simulink model "hybrid_system_diag"  (Simulink 7.8)
settings: Solver=FixedStepDiscrete  StartTime=0.0  StopTime=10  FixedStep=sim_sample_time  RelTol=1e-6
undefined symbols (not defined in the file or in its folder): SysHybride
settings Model: Creator=bayoudh  LastModifiedBy=szabi  ExtModeAutoUpdateStatusClock=off
settings OptimizationCC: InitFltsAndDblsToZero=on
settings DebuggingCC: SaveWithParameterizedLinksMsg=none  FcnCallInpInsideContextMsg=Use local settings  StrictBusMsg=Warning
settings SFSimCC: SimParseCustomCode=off
settings GRTTargetCC: TargetFcnLib=ansi_tfl_tmw.mat

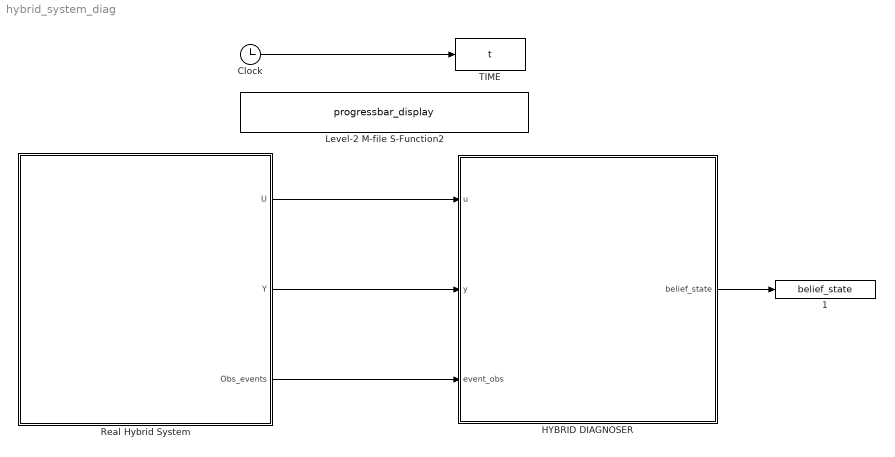
== system hybrid_system_diag ==
  1 : ToWorkspace  VariableName=belief_state  SampleTime=-1  SaveFormat=Array
  Clock : Clock
  "HYBRID DIAGNOSER " : Subsystem
  Level-2 M-file S-Function2 : M-S-Function  FunctionName=progressbar_display
  Real Hybrid System : Subsystem
  TIME : ToWorkspace  VariableName=t  SampleTime=-1  SaveFormat=Array
  wires:
  Clock/1 -> TIME/1
  Real Hybrid System/1(U) -> "HYBRID DIAGNOSER "/1(u)
  Real Hybrid System/2(Y) -> "HYBRID DIAGNOSER "/2(y)
  Real Hybrid System/3(Obs_events) -> "HYBRID DIAGNOSER "/3(event_obs)
  "HYBRID DIAGNOSER "/1(belief_state) -> 1/1

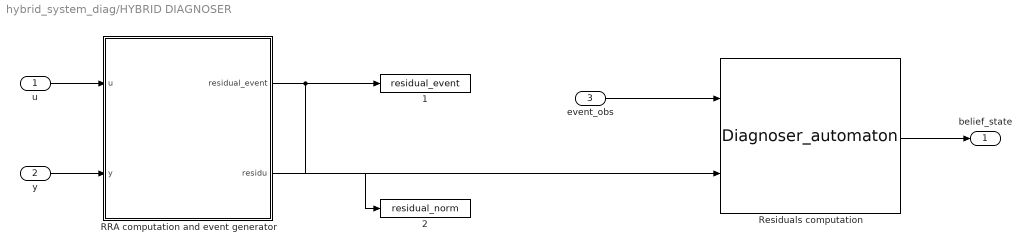
== system hybrid_system_diag/HYBRID DIAGNOSER  ==
  u : Inport
  y : Inport  Port=2
  event_obs : Inport  Port=3
  1 : ToWorkspace  VariableName=residual_event  SampleTime=-1  SaveFormat=Array
  2 : ToWorkspace  VariableName=residual_norm  SampleTime=-1  SaveFormat=Array
  RRA computation and event generator : Subsystem
  Residuals computation : M-S-Function  FunctionName=Diagnoser_automaton
  belief_state : Outport
  wires:
  u/1 -> RRA computation and event generator/1(u)
  y/1 -> RRA computation and event generator/2(y)
  RRA computation and event generator/1(residual_event) -> 1/1, Residuals computation/2
  RRA computation and event generator/2(residu) -> 2/1
  event_obs/1 -> Residuals computation/1
  Residuals computation/1 -> belief_state/1

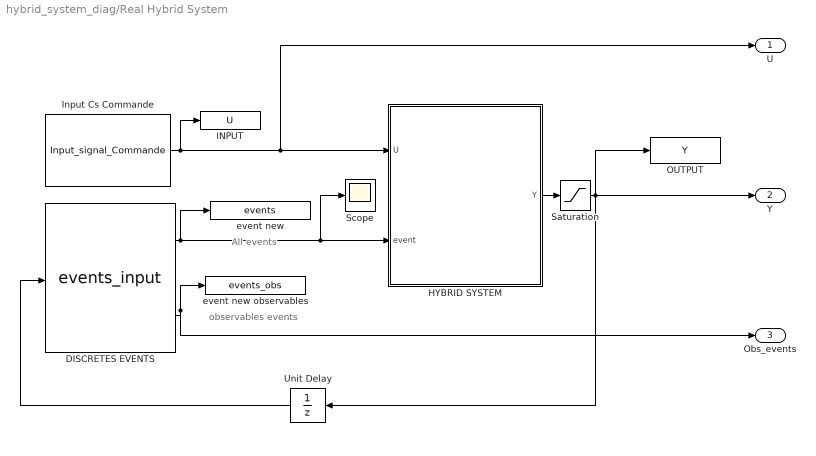
== system hybrid_system_diag/Real Hybrid System ==
  note: observables events
  note: All events
  DISCRETES EVENTS : M-S-Function  FunctionName=events_input
  HYBRID SYSTEM : Subsystem
  INPUT : ToWorkspace  VariableName=U  SampleTime=-1  SaveFormat=Array
  Input Cs Commande : S-Function  FunctionName=Input_signal_Commande  Parameters=rand(SysHybride('get_input_size'),1)*2*pi  EnableBusSupport=off
  OUTPUT : ToWorkspace  VariableName=Y  SampleTime=-1  SaveFormat=Array
  Saturation : Saturate  UpperLimit=Inf  LowerLimit=0
  Scope : Scope
  Unit Delay : UnitDelay  SampleTime=-1
  event new : ToWorkspace  VariableName=events  SampleTime=-1  SaveFormat=Array
  event new observables : ToWorkspace  VariableName=events_obs  SampleTime=-1  SaveFormat=Array
  U : Outport
  Y : Outport  Port=2
  Obs_events : Outport  Port=3
  wires:
  Input Cs Commande/1 -> INPUT/1, HYBRID SYSTEM/1(U), U/1
  HYBRID SYSTEM/1(Y) -> Saturation/1
  DISCRETES EVENTS/1 -> event new/1, HYBRID SYSTEM/2(event), Scope/1
  DISCRETES EVENTS/2 -> event new observables/1, Obs_events/1
  Unit Delay/1 -> DISCRETES EVENTS/1
  Saturation/1 -> Y/1, OUTPUT/1, Unit Delay/1

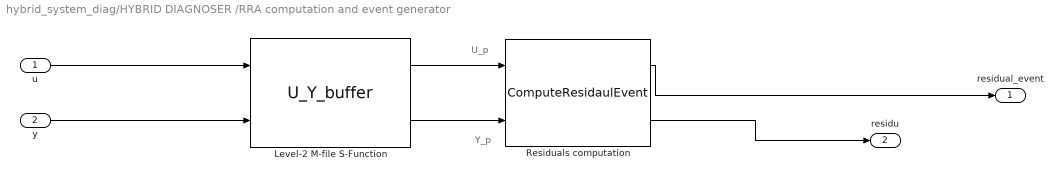
== system hybrid_system_diag/HYBRID DIAGNOSER /RRA computation and event generator ==
  note: U_p
  note: Y_p
  u : Inport
  y : Inport  Port=2
  Level-2 M-file S-Function : M-S-Function  FunctionName=U_Y_buffer
  Residuals computation : M-S-Function  FunctionName=ComputeResidaulEvent
  residual_event : Outport
  residu : Outport  Port=2
  wires:
  u/1 -> Level-2 M-file S-Function/1
  y/1 -> Level-2 M-file S-Function/2
  Level-2 M-file S-Function/1 -> Residuals computation/1
  Level-2 M-file S-Function/2 -> Residuals computation/2
  Residuals computation/1 -> residual_event/1
  Residuals computation/2 -> residu/1

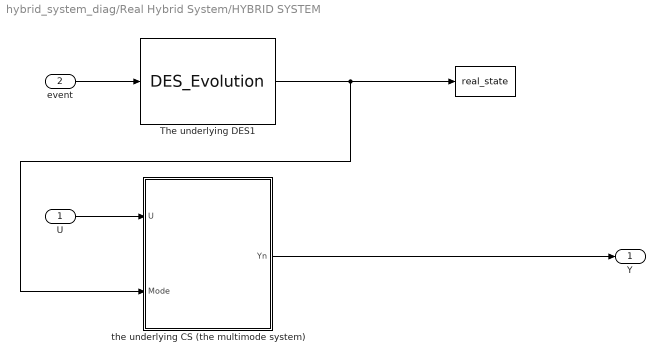
== system hybrid_system_diag/Real Hybrid System/HYBRID SYSTEM ==
  U : Inport
  event : Inport  Port=2
  "  " : ToWorkspace  VariableName=real_state  SampleTime=-1  SaveFormat=Array
  The underlying DES1 : S-Function  FunctionName=DES_Evolution  EnableBusSupport=off
  the underlying CS (the multimode system) : Subsystem
  Y : Outport
  wires:
  event/1 -> The underlying DES1/1
  U/1 -> the underlying CS (the multimode system)/1(U)
  The underlying DES1/1 -> the underlying CS (the multimode system)/2(Mode), "  "/1
  the underlying CS (the multimode system)/1(Yn) -> Y/1

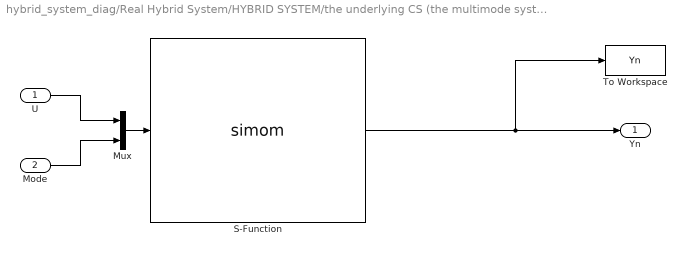
== system hybrid_system_diag/Real Hybrid System/HYBRID SYSTEM/the underlying CS (the multimode system) ==
  U : Inport
  Mode : Inport  Port=2
  Mux : Mux  Inputs=2
  S-Function : S-Function  FunctionName=simom  EnableBusSupport=off
  To Workspace : ToWorkspace  VariableName=Yn  SampleTime=-1  SaveFormat=Array
  Yn : Outport
  wires:
  S-Function/1 -> To Workspace/1, Yn/1
  U/1 -> Mux/1
  Mode/1 -> Mux/2
  Mux/1 -> S-Function/1
